simulink model "SF012A_HysCmp"  (R2013b)
settings: Solver=FixedStepDiscrete  StartTime=0.0  StopTime=1  FixedStep=.002  RelTol=1e-3
values from neighbouring files (symbols this model uses):
  ARCHGLBPRM_2MILLISEC_SEC_F32 = DataDict.Constant    [SF012A_HysCmp_DataDict.m]
  EPSILON_ULS_F32 = DataDict.Constant    [SF012A_HysCmp_DataDict.m]
  FLTINJ_HYSCMP_HYSCMPCMD = DataDict.Constant    [SF012A_HysCmp_DataDict.m]
  HysCmpAssiInpLim = DataDict.Calibration    [SF012A_HysCmp_DataDict.m]
  HysCmpOutpLim = DataDict.Calibration    [SF012A_HysCmp_DataDict.m]
  HysCmpRevGain = DataDict.Calibration    [SF012A_HysCmp_DataDict.m]
  HysCmpRiseX = DataDict.Calibration    [SF012A_HysCmp_DataDict.m]
  HysCmpRiseY = DataDict.Calibration    [SF012A_HysCmp_DataDict.m]
  HYSRISEYLIM_ULS_F32 = DataDict.Constant    [SF012A_HysCmp_DataDict.m]
  HYSSATNLOWLIM_HWNWTMTR_F32 = DataDict.Constant    [SF012A_HysCmp_DataDict.m]
  SysGlbPrmSysTqRat = DataDict.ImprtdCal    [SF012A_HysCmp_DataDict.m]
libraries: FixdToFloat x18, FloatToFixd x14, LnrIntrpn x12, NxtrAbslt x10, NxtrLim x8, Fil x6, NxtrSign x5, simulink x2, NxtrMath x1, BilnrIntrpnMplX x1, NxtrMax x1
(part 2 of 3)

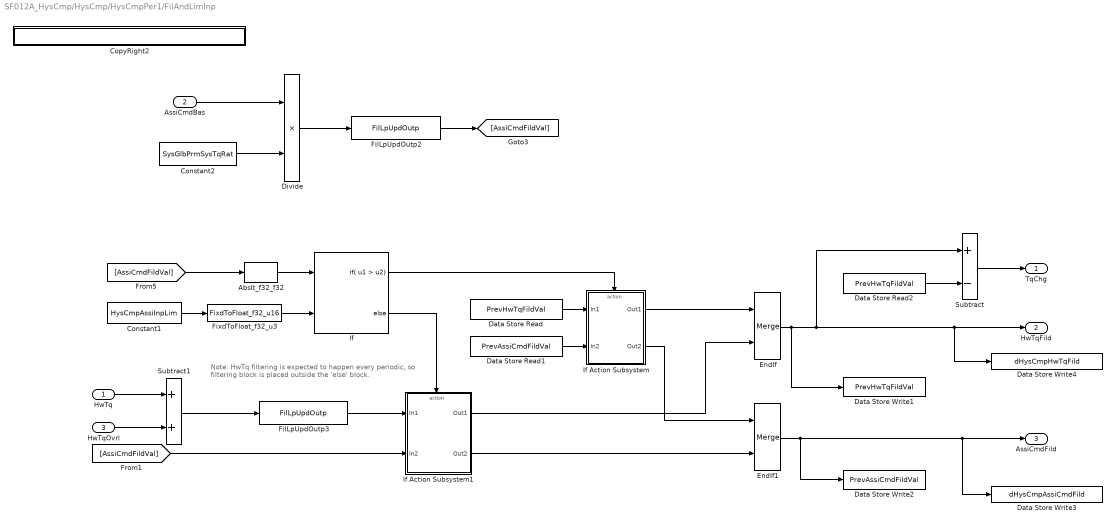
== system SF012A_HysCmp/HysCmp/HysCmpPer1/FilAndLimInp ==
  note: Note:
      | HwTq filtering is expected to happen every periodic, so filtering
      | block is placed outside the 'else' block.
  HwTq : Inport  RequirementInfo={'linktype_rmi_doors' '0000a52c (/E-STEER Core/SubSystem Specifications/Application Functions/SF012A Hysteresis Compensation)' '#SF012A_408' 'true' 'REQ:SF012A_408' '' } %GIDa_8595c692_04d6_4913_9dc2_51364eba2881
  AssiCmdBas : Inport  RequirementInfo={'linktype_rmi_doors' '0000a52c (/E-STEER Core/SubSystem Specifications/Application Functions/SF012A Hysteresis Compensation)' '#SF012A_409' 'true' 'REQ:SF012A_409' '' } %GIDa_dca39ed8_e3d9_4378_8b85_450d17c9d08c  Port=2
  HwTqOvrl : Inport  RequirementInfo={} %GIDa_e368a188_fa71_4a0d_b951_66914a67cd9f  Port=3
  Abslt_f32_f32 : NxtrAbslt/Abslt_f32_f32  RequirementInfo={'linktype_rmi_doors' '0000a52c (/E-STEER Core/SubSystem Specifications/Application Functions/SF012A Hysteresis Compensation)' '#SF012A_410' 'true' 'REQ:SF012A_410' '' ; 'linktype_rmi_doors' '0000a52c (/E-STEER Core/SubSystem Specifications/Application Functions/SF012A Hysteresis Compensation)' '#SF012A_411' 'true' 'REQ:SF012A_411' '' } %GIDa_f8d261e3_e868_420c_87ac_b2819908a7a3  SFunctionSpec=single y1 = Abslt_f32_f32(single u1)
      settings: AttributesFormatString=%<Name>
  Constant1 : Constant  RequirementInfo={'linktype_rmi_doors' '0000a52c (/E-STEER Core/SubSystem Specifications/Application Functions/SF012A Hysteresis Compensation)' '#SF012A_410' 'true' 'REQ:SF012A_410' '' ; 'linktype_rmi_doors' '0000a52c (/E-STEER Core/SubSystem Specifications/Application Functions/SF012A Hysteresis Compensation)' '#SF012A_411' 'true' 'REQ:SF012A_411' '' } %GIDa_864c3e61_20aa_4f8a_9abb_0e2225d86ec0  Value=HysCmpAssiInpLim
  Constant2 : Constant  RequirementInfo={'linktype_rmi_doors' '0000a52c (/E-STEER Core/SubSystem Specifications/Application Functions/SF012A Hysteresis Compensation)' '#SF012A_409' 'true' 'REQ:SF012A_409' '' } %GIDa_3b931750_8551_4b2a_8e8e_b917627f5aac  Value=SysGlbPrmSysTqRat
  CopyRight2 : Subsystem  Description=|  mask(Copyright Information){none=on}
      | Copyright info block.                                               
      |                                                                     
      | Place copyright information at the top of every subsystem in design.
      mask prompts: none "No parameters"
      mask help: Place copyright information at the top of every subsystem in design.
      mask Display:
      | NxtrConf = 'Nexteer Confidential';
      | 
      | sys = bdroot; %handle for the current model ("system")
      | first = get_param(sys,'Created');
      | if(isempty(first))
      |     first = datestr(now,'yyyy');
      | else
      |     first = first(end-3:end);  %year is last four digits
      | end
      | 
      | last = get_param(sys,'LastModifiedDate');
      | if isempty(last)
      |     last = datestr(now,'yyyy');
      | else
      |     last = last(end-3:end);
      | end
      | 
      | if strcmp(first,last)
      |     fprintf('%s -- Copyright %s Nexteer',NxtrConf,first)
      | else
      |     fprintf('%s -- %s%s- %s Nexteer',NxtrConf,char(169),first,last)
      | end
  Data Store Read : DataStoreRead  RequirementInfo={'linktype_rmi_doors' '0000a52c (/E-STEER Core/SubSystem Specifications/Application Functions/SF012A Hysteresis Compensation)' '#SF012A_410' 'true' 'REQ:SF012A_410' '' } %GIDa_fe2f0fc3_60a7_4f80_bf23_10f877f94ddf  DataStoreName=PrevHwTqFildVal
  Data Store Read1 : DataStoreRead  RequirementInfo={'linktype_rmi_doors' '0000a52c (/E-STEER Core/SubSystem Specifications/Application Functions/SF012A Hysteresis Compensation)' '#SF012A_411' 'true' 'REQ:SF012A_411' '' } %GIDa_d130b6b3_c629_46d9_812d_bdd319c1e1bb  DataStoreName=PrevAssiCmdFildVal
  Data Store Read2 : DataStoreRead  RequirementInfo={'linktype_rmi_doors' '0000a52c (/E-STEER Core/SubSystem Specifications/Application Functions/SF012A Hysteresis Compensation)' '#SF012A_413' 'true' 'REQ:SF012A_413' '' } %GIDa_ca0acc02_7cf7_474f_861e_05fd56275eb3  DataStoreName=PrevHwTqFildVal
  Data Store Write1 : DataStoreWrite  DataStoreName=PrevHwTqFildVal
  Data Store Write2 : DataStoreWrite  DataStoreName=PrevAssiCmdFildVal
  Data Store Write3 : DataStoreWrite  DataStoreName=dHysCmpAssiCmdFild
  Data Store Write4 : DataStoreWrite  DataStoreName=dHysCmpHwTqFild
  Divide : Product  RequirementInfo={'linktype_rmi_doors' '0000a52c (/E-STEER Core/SubSystem Specifications/Application Functions/SF012A Hysteresis Compensation)' '#SF012A_409' 'true' 'REQ:SF012A_409' '' } %GIDa_4801ace0_9cdb_47f1_b5c0_5f2abda0d87a
  EndIf : Merge
  EndIf1 : Merge
  FilLpUpdOutp2 : Fil/FilLpUpdOutp  RequirementInfo={'linktype_rmi_doors' '0000a52c (/E-STEER Core/SubSystem Specifications/Application Functions/SF012A Hysteresis Compensation)' '#SF012A_409' 'true' 'REQ:SF012A_409' '' } %GIDa_589584c9_b911_4f77_a83a_2b25e7b503c4  StVar=AssiCmdLpFil
      settings: AttributesFormatString=StVar: %<StVar>
  FilLpUpdOutp3 : Fil/FilLpUpdOutp  RequirementInfo={'linktype_rmi_doors' '0000a52c (/E-STEER Core/SubSystem Specifications/Application Functions/SF012A Hysteresis Compensation)' '#SF012A_408' 'true' 'REQ:SF012A_408' '' } %GIDa_7f89ab7f_0bec_4a90_b51d_fb631fff0f06  StVar=HwTqLpFil
      settings: AttributesFormatString=StVar: %<StVar>
  FixdToFloat_f32_u3 : FixdToFloat/FixdToFloat_f32_u16  RequirementInfo={'linktype_rmi_doors' '0000a52c (/E-STEER Core/SubSystem Specifications/Application Functions/SF012A Hysteresis Compensation)' '#SF012A_410' 'true' 'REQ:SF012A_410' '' ; 'linktype_rmi_doors' '0000a52c (/E-STEER Core/SubSystem Specifications/Application Functions/SF012A Hysteresis Compensation)' '#SF012A_411' 'true' 'REQ:SF012A_411' '' } %GIDa_0e35fb1f_9c33_4ae5_a8f9_936027a1a1ab  Param1=7
  If : If  RequirementInfo={'linktype_rmi_doors' '0000a52c (/E-STEER Core/SubSystem Specifications/Application Functions/SF012A Hysteresis Compensation)' '#SF012A_410' 'true' 'REQ:SF012A_410' '' ; 'linktype_rmi_doors' '0000a52c (/E-STEER Core/SubSystem Specifications/Application Functions/SF012A Hysteresis Compensation)' '#SF012A_411' 'true' 'REQ:SF012A_411' '' } %GIDa_f379a8d8_76cb_4a5a_bbf2_71e4ff64e958  NumInputs=2  IfExpression=u1 > u2
  If Action Subsystem : Subsystem  RequirementInfo={'linktype_rmi_doors' '0000a52c (/E-STEER Core/SubSystem Specifications/Application Functions/SF012A Hysteresis Compensation)' '#SF012A_410' 'true' 'REQ:SF012A_410' '' ; 'linktype_rmi_doors' '0000a52c (/E-STEER Core/SubSystem Specifications/Application Functions/SF012A Hysteresis Compensation)' '#SF012A_411' 'true' 'REQ:SF012A_411' '' } %GIDa_863f11eb_bed9_4787_8d86_71a303a919a1  TreatAsAtomicUnit=on
  If Action Subsystem1 : Subsystem  TreatAsAtomicUnit=on
  Subtract : Sum  RequirementInfo={'linktype_rmi_doors' '0000a52c (/E-STEER Core/SubSystem Specifications/Application Functions/SF012A Hysteresis Compensation)' '#SF012A_413' 'true' 'REQ:SF012A_413' '' } %GIDa_cc1a94d2_680b_41ba_bf31_9725f502d028  Inputs=+-  RndMeth=Zero
  Subtract1 : Sum  RequirementInfo="{'linktype_rmi_doors' '0000a52c (/E-STEER Core/SubSystem Specifications/Application Functions/SF012A Hysteresis Compensation)' '#SF012A_413' 'true' 'REQ:SF012A_413' '' ; 'linktype_rmi_doors' '0000a52c (/E-STEER Core/SubSystem Specifications/Application Functions/SF012A Hysteresis Compensation)' '#SF012A_408' 'true' 'REQ:  SF012A_408' '' } %GIDa_c73f89c5_e69d_4c2f_8313_728af91665f8"  RndMeth=Zero
  TqChg : Outport  RequirementInfo={'linktype_rmi_doors' '0000a52c (/E-STEER Core/SubSystem Specifications/Application Functions/SF012A Hysteresis Compensation)' '#SF012A_412' 'true' 'REQ:SF012A_412' '' } %GIDa_bba798dc_3c8f_457b_9533_3f83bd880396
  HwTqFild : Outport  Port=2
  AssiCmdFild : Outport  Port=3
  wires:
  FilLpUpdOutp2/1 -> [AssiCmdFildVal]
  Divide/1 -> FilLpUpdOutp2/1
  AssiCmdBas/1 -> Divide/1
  Constant2/1 -> Divide/2
  [AssiCmdFildVal] -> Abslt_f32_f32/1
  Abslt_f32_f32/1 -> If/1
  Constant1/1 -> FixdToFloat_f32_u3/1
  If/1 -> If Action Subsystem/Action
  If/2 -> If Action Subsystem1/Action
  [AssiCmdFildVal] -> If Action Subsystem1/2(In2)
  FilLpUpdOutp3/1 -> If Action Subsystem1/1(In1)
  If Action Subsystem1/1(Out1) -> EndIf/2
  If Action Subsystem/1(Out1) -> EndIf/1
  Data Store Read/1 -> If Action Subsystem/1(In1)
  Data Store Read1/1 -> If Action Subsystem/2(In2)
  If Action Subsystem/2(Out2) -> EndIf1/1
  If Action Subsystem1/2(Out2) -> EndIf1/2
  Subtract/1 -> TqChg/1
  EndIf/1 -> Data Store Write1/1, Data Store Write4/1, HwTqFild/1, Subtract/1
  Data Store Read2/1 -> Subtract/2
  EndIf1/1 -> Data Store Write3/1, AssiCmdFild/1, Data Store Write2/1
  FixdToFloat_f32_u3/1 -> If/2
  Subtract1/1 -> FilLpUpdOutp3/1
  HwTq/1 -> Subtract1/1
  HwTqOvrl/1 -> Subtract1/2

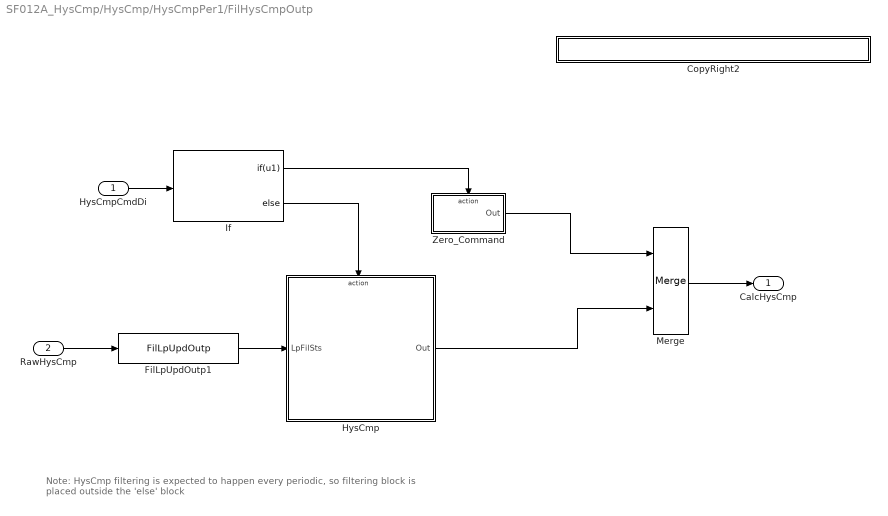
== system SF012A_HysCmp/HysCmp/HysCmpPer1/FilHysCmpOutp ==
  note: Note:
      | HysCmp filtering is expected to happen every periodic, so filtering block is placed
      | outside the 'else' block
  HysCmpCmdDi : Inport  RequirementInfo={'linktype_rmi_doors' '0000a52c (/E-STEER Core/SubSystem Specifications/Application Functions/SF012A Hysteresis Compensation)' '#SF012A_459' 'true' 'REQ:SF012A_459' '' } %GIDa_23db5d3c_8a57_4504_bba3_7c9578b077b2
  RawHysCmp : Inport  RequirementInfo={'linktype_rmi_doors' '0000a52c (/E-STEER Core/SubSystem Specifications/Application Functions/SF012A Hysteresis Compensation)' '#SF012A_457' 'true' 'REQ:SF012A_457' '' } %GIDa_195e1d1d_69bd_4591_afc7_b0c2a9192583  Port=2
  CopyRight2 : Subsystem  Description=|  mask(Copyright Information){none=on}
      | Copyright info block.                                               
      |                                                                     
      | Place copyright information at the top of every subsystem in design.
      mask prompts: none "No parameters"
      mask help: Place copyright information at the top of every subsystem in design.
      mask Display:
      | NxtrConf = 'Nexteer Confidential';
      | 
      | sys = bdroot; %handle for the current model ("system")
      | first = get_param(sys,'Created');
      | if(isempty(first))
      |     first = datestr(now,'yyyy');
      | else
      |     first = first(end-3:end);  %year is last four digits
      | end
      | 
      | last = get_param(sys,'LastModifiedDate');
      | if isempty(last)
      |     last = datestr(now,'yyyy');
      | else
      |     last = last(end-3:end);
      | end
      | 
      | if strcmp(first,last)
      |     fprintf('%s -- Copyright %s Nexteer',NxtrConf,first)
      | else
      |     fprintf('%s -- %s%s- %s Nexteer',NxtrConf,char(169),first,last)
      | end
  FilLpUpdOutp1 : Fil/FilLpUpdOutp  RequirementInfo={'linktype_rmi_doors' '0000a52c (/E-STEER Core/SubSystem Specifications/Application Functions/SF012A Hysteresis Compensation)' '#SF012A_457' 'true' 'REQ:SF012A_457' '' } %GIDa_9e2ef691_d79e_479f_a90d_387920e70bae  StVar=FinalOutpLpFil
      settings: AttributesFormatString=StVar: %<StVar>
  HysCmp : Subsystem  RequirementInfo={} %GIDa_95224ba3_d373_47aa_9e2d_c8f1beaf79f1  TreatAsAtomicUnit=on
  If : If  RequirementInfo={'linktype_rmi_doors' '0000a52c (/E-STEER Core/SubSystem Specifications/Application Functions/SF012A Hysteresis Compensation)' '#SF012A_459' 'true' 'REQ:SF012A_459' '' } %GIDa_94a310f4_6e32_4cd6_8e0d_2a7931f46409  IfExpression=u1
  Merge : Merge
  Zero_Command : Subsystem  RequirementInfo={'linktype_rmi_doors' '0000a52c (/E-STEER Core/SubSystem Specifications/Application Functions/SF012A Hysteresis Compensation)' '#SF012A_459' 'true' 'REQ:SF012A_459' '' } %GIDa_7dfea39b_76f9_4579_a42d_48172b08e8b5  TreatAsAtomicUnit=on
  CalcHysCmp : Outport
  wires:
  HysCmp/1(Out) -> Merge/2
  If/1 -> Zero_Command/Action
  If/2 -> HysCmp/Action
  HysCmpCmdDi/1 -> If/1
  Zero_Command/1(Out) -> Merge/1
  Merge/1 -> CalcHysCmp/1
  RawHysCmp/1 -> FilLpUpdOutp1/1
  FilLpUpdOutp1/1 -> HysCmp/1(LpFilSts)

== system SF012A_HysCmp/HysCmp/HysCmpPer1/FltInj - Sim ==
  note: Inport #2 must be Constant
  note: EA4.x Fault Injection
  note: This block requires no modification by FDD author.
      |
      | This block does not actually simulate any fault injection.  It is simply a pass-thru.
      |
      | The port (#2) simply terminates its signal, but we are trying to force the FDD author
      | to properly use the Constant in FDD model.
  HysCmp : Inport
  FltInjCon : Inport  Port=2
  CopyRight2 : Subsystem  Description=|  mask(Copyright Information){none=on}
      | Copyright info block.                                               
      |                                                                     
      | Place copyright information at the top of every subsystem in design.
      mask prompts: none "No parameters"
      mask help: Place copyright information at the top of every subsystem in design.
      mask Display:
      | NxtrConf = 'Nexteer Confidential';
      | 
      | sys = bdroot; %handle for the current model ("system")
      | first = get_param(sys,'Created');
      | if(isempty(first))
      |     first = datestr(now,'yyyy');
      | else
      |     first = first(end-3:end);  %year is last four digits
      | end
      | 
      | last = get_param(sys,'LastModifiedDate');
      | if isempty(last)
      |     last = datestr(now,'yyyy');
      | else
      |     last = last(end-3:end);
      | end
      | 
      | if strcmp(first,last)
      |     fprintf('%s -- Copyright %s Nexteer',NxtrConf,first)
      | else
      |     fprintf('%s -- %s%s- %s Nexteer',NxtrConf,char(169),first,last)
      | end
  Terminator : Terminator
  Outp : Outport
  wires:
  FltInjCon/1 -> Terminator/1
  HysCmp/1 -> Outp/1

== system SF012A_HysCmp/HysCmp/HysCmpPer1/CalcAvlCmp/CopyRight2 ==

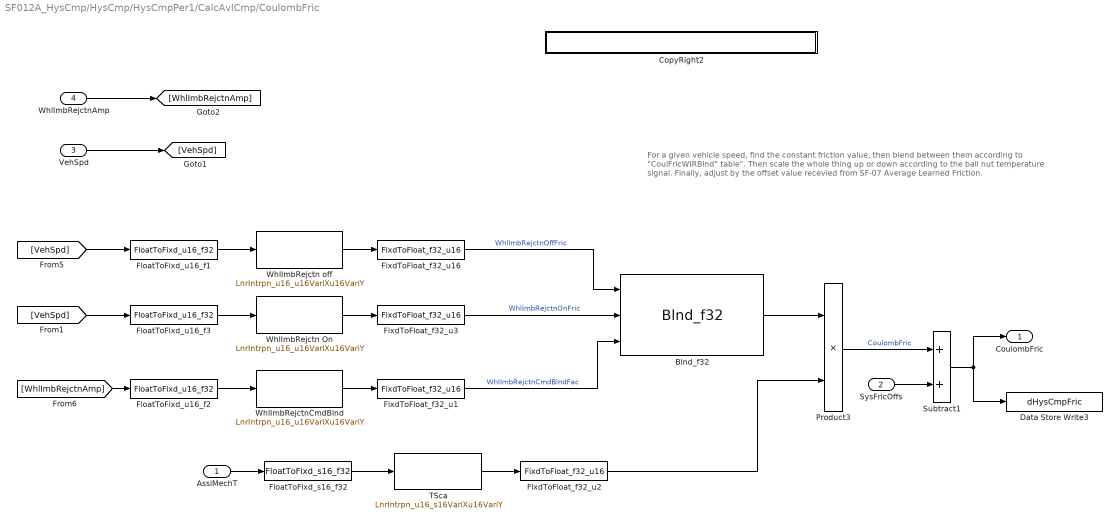
== system SF012A_HysCmp/HysCmp/HysCmpPer1/CalcAvlCmp/CoulombFric ==
  note: For a given vehicle speed, find the constant friction value, then blend between them
      | according to "CoulFricWIRBlnd" table".
      |
      | Then scale the whole thing up or down according to the ball nut temperature signal.
      |
      | Finally, adjust by the offset value recevied from SF-07 Average Learned Friction.
  AssiMechT : Inport  RequirementInfo={'linktype_rmi_doors' '0000a52c (/E-STEER Core/SubSystem Specifications/Application Functions/SF012A Hysteresis Compensation)' '#SF012A_449' 'true' 'REQ:SF012A_449' '' } %GIDa_99e06030_f9cc_4e47_87aa_b53708a11645
  SysFricOffs : Inport  RequirementInfo={'linktype_rmi_doors' '0000a52c (/E-STEER Core/SubSystem Specifications/Application Functions/SF012A Hysteresis Compensation)' '#SF012A_450' 'true' 'REQ:SF012A_450' '' } %GIDa_ac543b49_7806_48b8_bba0_d91827b9781a  Port=2
  VehSpd : Inport  Port=3
  WhlImbRejctnAmp : Inport  Port=4
  Blnd_f32 : NxtrMath/Blnd_f32  RequirementInfo={'linktype_rmi_doors' '0000a52c (/E-STEER Core/SubSystem Specifications/Application Functions/SF012A Hysteresis Compensation)' '#SF012A_448' 'true' 'REQ:SF012A_448' '' } %GIDa_bbdb4f9c_3bc2_498f_af71_2f49518b1990  SFunctionSpec=single y1 = Blnd_f32(single u1, single u2, single u3)  Parameter3=on
      settings: AttributesFormatString=%<Name>
  CopyRight2 : Subsystem  Description=|  mask(Copyright Information){none=on}
      | Copyright info block.                                               
      |                                                                     
      | Place copyright information at the top of every subsystem in design.
      mask prompts: none "No parameters"
      mask help: Place copyright information at the top of every subsystem in design.
      mask Display:
      | NxtrConf = 'Nexteer Confidential';
      | 
      | sys = bdroot; %handle for the current model ("system")
      | first = get_param(sys,'Created');
      | if(isempty(first))
      |     first = datestr(now,'yyyy');
      | else
      |     first = first(end-3:end);  %year is last four digits
      | end
      | 
      | last = get_param(sys,'LastModifiedDate');
      | if isempty(last)
      |     last = datestr(now,'yyyy');
      | else
      |     last = last(end-3:end);
      | end
      | 
      | if strcmp(first,last)
      |     fprintf('%s -- Copyright %s Nexteer',NxtrConf,first)
      | else
      |     fprintf('%s -- %s%s- %s Nexteer',NxtrConf,char(169),first,last)
      | end
  Data Store Write3 : DataStoreWrite  RequirementInfo={'linktype_rmi_doors' '0000a52c (/E-STEER Core/SubSystem Specifications/Application Functions/SF012A Hysteresis Compensation)' '#SF012A_450' 'true' 'REQ:SF012A_450' '' } %GIDa_6d45951a_d82c_43e3_9e30_495c6992e5fa  DataStoreName=dHysCmpFric
  FixdToFloat_f32_u1 : FixdToFloat/FixdToFloat_f32_u16  RequirementInfo={'linktype_rmi_doors' '0000a52c (/E-STEER Core/SubSystem Specifications/Application Functions/SF012A Hysteresis Compensation)' '#SF012A_447' 'true' 'REQ:SF012A_447' '' } %GIDa_6923d4d2_9d71_4e52_940a_040d870df5d3  Param1=14
  FixdToFloat_f32_u16 : FixdToFloat/FixdToFloat_f32_u16  RequirementInfo={'linktype_rmi_doors' '0000a52c (/E-STEER Core/SubSystem Specifications/Application Functions/SF012A Hysteresis Compensation)' '#SF012A_445' 'true' 'REQ:SF012A_445' '' } %GIDa_30d19d68_5b37_4b98_9d06_6ac023f5c633  Param1=7
  FixdToFloat_f32_u2 : FixdToFloat/FixdToFloat_f32_u16  RequirementInfo={'linktype_rmi_doors' '0000a52c (/E-STEER Core/SubSystem Specifications/Application Functions/SF012A Hysteresis Compensation)' '#SF012A_449' 'true' 'REQ:SF012A_449' '' } %GIDa_e9926a9e_58d8_4e0f_b85f_c8f228f08a51  Param1=7
  FixdToFloat_f32_u3 : FixdToFloat/FixdToFloat_f32_u16  RequirementInfo={'linktype_rmi_doors' '0000a52c (/E-STEER Core/SubSystem Specifications/Application Functions/SF012A Hysteresis Compensation)' '#SF012A_446' 'true' 'REQ:SF012A_446' '' } %GIDa_029b97c1_98e5_43d6_8bb2_f228e7ba74a0  Param1=7
  FloatToFixd_s16_f32 : FloatToFixd/FloatToFixd_s16_f32  RequirementInfo={'linktype_rmi_doors' '0000a52c (/E-STEER Core/SubSystem Specifications/Application Functions/SF012A Hysteresis Compensation)' '#SF012A_449' 'true' 'REQ:SF012A_449' '' } %GIDa_ed7de31a_137c_4cee_b956_f1a1d053aab7  Param1=1
  FloatToFixd_u16_f1 : FloatToFixd/FloatToFixd_u16_f32  RequirementInfo={'linktype_rmi_doors' '0000a52c (/E-STEER Core/SubSystem Specifications/Application Functions/SF012A Hysteresis Compensation)' '#SF012A_445' 'true' 'REQ:SF012A_445' '' } %GIDa_d5c90da9_066a_4c50_b363_eaa13c485fc7  Param1=7
  FloatToFixd_u16_f2 : FloatToFixd/FloatToFixd_u16_f32  RequirementInfo={'linktype_rmi_doors' '0000a52c (/E-STEER Core/SubSystem Specifications/Application Functions/SF012A Hysteresis Compensation)' '#SF012A_447' 'true' 'REQ:SF012A_447' '' } %GIDa_1211a0db_eafe_40ef_b441_39a05294fb9a  Param1=8
  FloatToFixd_u16_f3 : FloatToFixd/FloatToFixd_u16_f32  RequirementInfo={'linktype_rmi_doors' '0000a52c (/E-STEER Core/SubSystem Specifications/Application Functions/SF012A Hysteresis Compensation)' '#SF012A_446' 'true' 'REQ:SF012A_446' '' } %GIDa_1e28c5e9_2e43_4a13_a086_2e913b05aeaf  Param1=7
  Product3 : Product  RequirementInfo={'linktype_rmi_doors' '0000a52c (/E-STEER Core/SubSystem Specifications/Application Functions/SF012A Hysteresis Compensation)' '#SF012A_449' 'true' 'REQ:SF012A_449' '' } %GIDa_88ab9335_d857_42a9_939b_fda1c9a4430d  RndMeth=Zero
  Subtract1 : Sum  RequirementInfo={'linktype_rmi_doors' '0000a52c (/E-STEER Core/SubSystem Specifications/Application Functions/SF012A Hysteresis Compensation)' '#SF012A_450' 'true' 'REQ:SF012A_450' '' } %GIDa_00ed35e3_2a2d_45e4_ac36_bcf0983ee021
  TSca : LnrIntrpn/LnrIntrpn_u16_s16VariXu16VariY  RequirementInfo={'linktype_rmi_doors' '0000a52c (/E-STEER Core/SubSystem Specifications/Application Functions/SF012A Hysteresis Compensation)' '#SF012A_449' 'true' 'REQ:SF012A_449' '' } %GIDa_1507d625_50ab_420f_903c_b0ff65633902  XTbl=HysCmpFricTScaX  YTbl=HysCmpFricTScaY
      settings: AttributesFormatString=Lnr ( s16VariX , u16VariY )
  WhlImbRejctn On : LnrIntrpn/LnrIntrpn_u16_u16VariXu16VariY  RequirementInfo={'linktype_rmi_doors' '0000a52c (/E-STEER Core/SubSystem Specifications/Application Functions/SF012A Hysteresis Compensation)' '#SF012A_446' 'true' 'REQ:SF012A_446' '' } %GIDa_3da3a5f4_48bb_4b0e_875e_441bf1ad5aca  XTbl=SysGlbPrmVehSpdBilnrSeln  YTbl=HysCmpFricWhlImbRejctnOnY
      settings: AttributesFormatString=Lnr ( u16VariX , u16VariY )
  WhlImbRejctn off : LnrIntrpn/LnrIntrpn_u16_u16VariXu16VariY  RequirementInfo={'linktype_rmi_doors' '0000a52c (/E-STEER Core/SubSystem Specifications/Application Functions/SF012A Hysteresis Compensation)' '#SF012A_445' 'true' 'REQ:SF012A_445' '' } %GIDa_4a3d582a_5707_4fce_81eb_d8533e9ef487  XTbl=SysGlbPrmVehSpdBilnrSeln  YTbl=HysCmpFricWhlImbRejctnOffY
      settings: AttributesFormatString=Lnr ( u16VariX , u16VariY )
  WhlImbRejctnCmdBlnd : LnrIntrpn/LnrIntrpn_u16_u16VariXu16VariY  RequirementInfo={'linktype_rmi_doors' '0000a52c (/E-STEER Core/SubSystem Specifications/Application Functions/SF012A Hysteresis Compensation)' '#SF012A_447' 'true' 'REQ:SF012A_447' '' } %GIDa_665c52af_bd47_42fe_9c42_9c84618a0bfd  XTbl=HysCmpFricWhlImbRejctnBlndX  YTbl=HysCmpFricWhlImbRejctnBlndY
      settings: AttributesFormatString=Lnr ( u16VariX , u16VariY )
  CoulombFric : Outport  RequirementInfo={'linktype_rmi_doors' '0000a52c (/E-STEER Core/SubSystem Specifications/Application Functions/SF012A Hysteresis Compensation)' '#SF012A_450' 'true' 'REQ:SF012A_450' '' } %GIDa_05ee5a21_5232_467a_82a3_6197e6a6ac48
  wires:
  AssiMechT/1 -> FloatToFixd_s16_f32/1
  SysFricOffs/1 -> Subtract1/2
  VehSpd/1 -> [VehSpd]
  WhlImbRejctnAmp/1 -> [WhlImbRejctnAmp]
  FloatToFixd_s16_f32/1 -> TSca/1
  TSca/1 -> FixdToFloat_f32_u2/1
  FixdToFloat_f32_u2/1 -> Product3/2
  Product3/1 -> Subtract1/1  "CoulombFric"
  Subtract1/1 -> Data Store Write3/1, CoulombFric/1
  [VehSpd] -> FloatToFixd_u16_f1/1
  FloatToFixd_u16_f1/1 -> WhlImbRejctn off/1
  WhlImbRejctnCmdBlnd/1 -> FixdToFloat_f32_u1/1
  [WhlImbRejctnAmp] -> FloatToFixd_u16_f2/1
  FixdToFloat_f32_u16/1 -> Blnd_f32/1  "WhlImbRejctnOffFric"
  FloatToFixd_u16_f2/1 -> WhlImbRejctnCmdBlnd/1
  FixdToFloat_f32_u1/1 -> Blnd_f32/3  "WhlImbRejctnCmdBlndFac"
  [VehSpd] -> FloatToFixd_u16_f3/1
  FloatToFixd_u16_f3/1 -> WhlImbRejctn On/1
  FixdToFloat_f32_u3/1 -> Blnd_f32/2  "WhlImbRejctnOnFric"
  WhlImbRejctn On/1 -> FixdToFloat_f32_u3/1
  WhlImbRejctn off/1 -> FixdToFloat_f32_u16/1
  Blnd_f32/1 -> Product3/1

== system SF012A_HysCmp/HysCmp/HysCmpPer1/CalcRiseFac/CopyRight2 ==

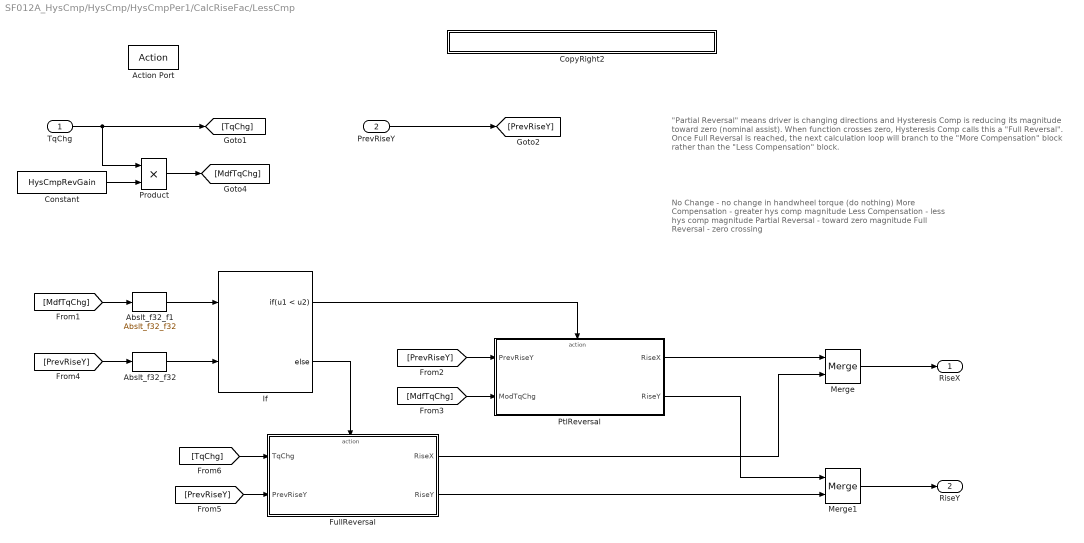
== system SF012A_HysCmp/HysCmp/HysCmpPer1/CalcRiseFac/LessCmp ==
  note: No Change                    - no change in handwheel torque (do nothing)
      |
      | More Compensation     - greater hys comp magnitude
      |
      | Less Compensation     - less hys comp magnitude
      |        Partial Reversal          - toward zero magnitude
      |        Full Reversal               - zero crossing
  note: "Partial Reversal" means driver is changing directions and Hysteresis Comp is reducing its magnitude toward
      | zero (nominal assist).  When function crosses zero, Hysteresis Comp calls this a "Full Reversal".  Once
      | Full Reversal is reached, the next calculation loop will branch to the "More Compensation" block rather
      | than the "Less Compensation" block.
  TqChg : Inport  RequirementInfo={'linktype_rmi_doors' '0000a52c (/E-STEER Core/SubSystem Specifications/Application Functions/SF012A Hysteresis Compensation)' '#SF012A_427' 'true' 'REQ:SF012A_427' '' } %GIDa_99dd5ad1_f987_430b_9292_ba160c7a64e2
  PrevRiseY : Inport  Port=2
  Action Port : ActionPort  ActionType=else
  Abslt_f32_f1 : NxtrAbslt/Abslt_f32_f32  RequirementInfo={'linktype_rmi_doors' '0000a52c (/E-STEER Core/SubSystem Specifications/Application Functions/SF012A Hysteresis Compensation)' '#SF012A_430' 'true' 'REQ:SF012A_430' '' ; 'linktype_rmi_doors' '0000a52c (/E-STEER Core/SubSystem Specifications/Application Functions/SF012A Hysteresis Compensation)' '#SF012A_434' 'true' 'REQ:SF012A_434' '' } %GIDa_cb35d4e0_44c4_4ae0_8e61_ff94531bb974  SFunctionSpec=single y1 = Abslt_f32_f32(single u1)
      settings: AttributesFormatString=%<Name>
  Abslt_f32_f32 : NxtrAbslt/Abslt_f32_f32  RequirementInfo={'linktype_rmi_doors' '0000a52c (/E-STEER Core/SubSystem Specifications/Application Functions/SF012A Hysteresis Compensation)' '#SF012A_430' 'true' 'REQ:SF012A_430' '' ; 'linktype_rmi_doors' '0000a52c (/E-STEER Core/SubSystem Specifications/Application Functions/SF012A Hysteresis Compensation)' '#SF012A_434' 'true' 'REQ:SF012A_434' '' } %GIDa_784ab8b6_4235_4986_832e_173db3fc1314  SFunctionSpec=single y1 = Abslt_f32_f32(single u1)
      settings: AttributesFormatString=%<Name>
  Constant : Constant  RequirementInfo={'linktype_rmi_doors' '0000a52c (/E-STEER Core/SubSystem Specifications/Application Functions/SF012A Hysteresis Compensation)' '#SF012A_427' 'true' 'REQ:SF012A_427' '' } %GIDa_15f6df37_2f5f_4b2b_9a59_ced4ab5b144b  Value=HysCmpRevGain
  CopyRight2 : Subsystem  Description=|  mask(Copyright Information){none=on}
      | Copyright info block.                                               
      |                                                                     
      | Place copyright information at the top of every subsystem in design.
      mask prompts: none "No parameters"
      mask help: Place copyright information at the top of every subsystem in design.
      mask Display:
      | NxtrConf = 'Nexteer Confidential';
      | 
      | sys = bdroot; %handle for the current model ("system")
      | first = get_param(sys,'Created');
      | if(isempty(first))
      |     first = datestr(now,'yyyy');
      | else
      |     first = first(end-3:end);  %year is last four digits
      | end
      | 
      | last = get_param(sys,'LastModifiedDate');
      | if isempty(last)
      |     last = datestr(now,'yyyy');
      | else
      |     last = last(end-3:end);
      | end
      | 
      | if strcmp(first,last)
      |     fprintf('%s -- Copyright %s Nexteer',NxtrConf,first)
      | else
      |     fprintf('%s -- %s%s- %s Nexteer',NxtrConf,char(169),first,last)
      | end
  FullReversal : Subsystem  RequirementInfo={'linktype_rmi_doors' '0000a52c (/E-STEER Core/SubSystem Specifications/Application Functions/SF012A Hysteresis Compensation)' '#SF012A_433' 'true' 'REQ:SF012A_433' '' } %GIDa_ec6c7e68_d561_42f7_b642_302ca9573c52  TreatAsAtomicUnit=on
  If : If  RequirementInfo={'linktype_rmi_doors' '0000a52c (/E-STEER Core/SubSystem Specifications/Application Functions/SF012A Hysteresis Compensation)' '#SF012A_430' 'true' 'REQ:SF012A_430' '' ; 'linktype_rmi_doors' '0000a52c (/E-STEER Core/SubSystem Specifications/Application Functions/SF012A Hysteresis Compensation)' '#SF012A_434' 'true' 'REQ:SF012A_434' '' } %GIDa_cd0f389b_ef71_46b6_bbe9_7b7e3cd1952a  NumInputs=2  IfExpression=u1 < u2
  Merge : Merge
  Merge1 : Merge
  Product : Product  RequirementInfo={'linktype_rmi_doors' '0000a52c (/E-STEER Core/SubSystem Specifications/Application Functions/SF012A Hysteresis Compensation)' '#SF012A_427' 'true' 'REQ:SF012A_427' '' } %GIDa_7ff331fe_9280_41b2_bd53_ab63015d89f2  RndMeth=Zero
  PtlReversal : Subsystem  RequirementInfo={'linktype_rmi_doors' '0000a52c (/E-STEER Core/SubSystem Specifications/Application Functions/SF012A Hysteresis Compensation)' '#SF012A_429' 'true' 'REQ:SF012A_429' '' } %GIDa_b76a0e39_afe4_4599_8d0e_a01df819218b  TreatAsAtomicUnit=on
  RiseX : Outport
  RiseY : Outport  Port=2
  wires:
  TqChg/1 -> Product/1, [TqChg]
  PrevRiseY/1 -> [PrevRiseY]
  Product/1 -> [MdfTqChg]
  [PrevRiseY] -> Abslt_f32_f32/1
  Abslt_f32_f32/1 -> If/2
  [MdfTqChg] -> Abslt_f32_f1/1
  Abslt_f32_f1/1 -> If/1
  If/1 -> PtlReversal/Action
  If/2 -> FullReversal/Action
  [PrevRiseY] -> PtlReversal/1(PrevRiseY)
  [MdfTqChg] -> PtlReversal/2(ModTqChg)
  [PrevRiseY] -> FullReversal/2(PrevRiseY)
  [TqChg] -> FullReversal/1(TqChg)
  PtlReversal/1(RiseX) -> Merge/1
  PtlReversal/2(RiseY) -> Merge1/1
  Merge/1 -> RiseX/1
  Merge1/1 -> RiseY/1
  FullReversal/1(RiseX) -> Merge/2
  FullReversal/2(RiseY) -> Merge1/2
  Constant/1 -> Product/2

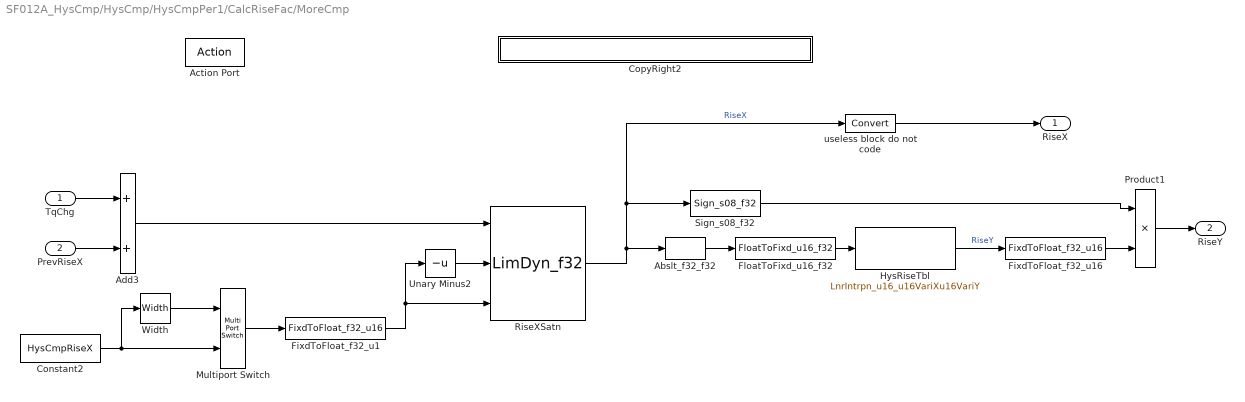
== system SF012A_HysCmp/HysCmp/HysCmpPer1/CalcRiseFac/MoreCmp ==
  TqChg : Inport  RequirementInfo={'linktype_rmi_doors' '0000a52c (/E-STEER Core/SubSystem Specifications/Application Functions/SF012A Hysteresis Compensation)' '#SF012A_423' 'true' 'REQ:SF012A_423' '' } %GIDa_dcd955d8_e60c_4b32_934a_4c581dd85aa1
  PrevRiseX : Inport  RequirementInfo={'linktype_rmi_doors' '0000a52c (/E-STEER Core/SubSystem Specifications/Application Functions/SF012A Hysteresis Compensation)' '#SF012A_423' 'true' 'REQ:SF012A_423' '' } %GIDa_087dae41_8153_4d25_bd8f_934a3a8ff619  Port=2
  Action Port : ActionPort  ActionType=elseif
  Abslt_f32_f32 : NxtrAbslt/Abslt_f32_f32  RequirementInfo={'linktype_rmi_doors' '0000a52c (/E-STEER Core/SubSystem Specifications/Application Functions/SF012A Hysteresis Compensation)' '#SF012A_425' 'true' 'REQ:SF012A_425' '' } %GIDa_32c7f8a9_d2f9_4a69_a73d_851dc6a3d9da  SFunctionSpec=single y1 = Abslt_f32_f32(single u1)
      settings: AttributesFormatString=%<Name>
  Add3 : Sum  RequirementInfo={'linktype_rmi_doors' '0000a52c (/E-STEER Core/SubSystem Specifications/Application Functions/SF012A Hysteresis Compensation)' '#SF012A_423' 'true' 'REQ:SF012A_423' '' } %GIDa_d9459225_db2d_4211_a8e1_86c473c2aa48  RndMeth=Zero
  Constant2 : Constant  RequirementInfo={'linktype_rmi_doors' '0000a52c (/E-STEER Core/SubSystem Specifications/Application Functions/SF012A Hysteresis Compensation)' '#SF012A_424' 'true' 'REQ:SF012A_424' '' } %GIDa_d2b201c3_0390_42ff_a153_be580eaf717d  Value=HysCmpRiseX
  CopyRight2 : Subsystem  Description=|  mask(Copyright Information){none=on}
      | Copyright info block.                                               
      |                                                                     
      | Place copyright information at the top of every subsystem in design.
      mask prompts: none "No parameters"
      mask help: Place copyright information at the top of every subsystem in design.
      mask Display:
      | NxtrConf = 'Nexteer Confidential';
      | 
      | sys = bdroot; %handle for the current model ("system")
      | first = get_param(sys,'Created');
      | if(isempty(first))
      |     first = datestr(now,'yyyy');
      | else
      |     first = first(end-3:end);  %year is last four digits
      | end
      | 
      | last = get_param(sys,'LastModifiedDate');
      | if isempty(last)
      |     last = datestr(now,'yyyy');
      | else
      |     last = last(end-3:end);
      | end
      | 
      | if strcmp(first,last)
      |     fprintf('%s -- Copyright %s Nexteer',NxtrConf,first)
      | else
      |     fprintf('%s -- %s%s- %s Nexteer',NxtrConf,char(169),first,last)
      | end
  FixdToFloat_f32_u1 : FixdToFloat/FixdToFloat_f32_u16  RequirementInfo={'linktype_rmi_doors' '0000a52c (/E-STEER Core/SubSystem Specifications/Application Functions/SF012A Hysteresis Compensation)' '#SF012A_424' 'true' 'REQ:SF012A_424' '' } %GIDa_ba8154cf_569f_4ec9_bec9_04076a244e06  Param1=14
  FixdToFloat_f32_u16 : FixdToFloat/FixdToFloat_f32_u16  RequirementInfo={'linktype_rmi_doors' '0000a52c (/E-STEER Core/SubSystem Specifications/Application Functions/SF012A Hysteresis Compensation)' '#SF012A_425' 'true' 'REQ:SF012A_425' '' } %GIDa_9bb57ca1_48e0_4f1a_9eca_c1d1a458fd1d  Param1=14
  FloatToFixd_u16_f32 : FloatToFixd/FloatToFixd_u16_f32  RequirementInfo={'linktype_rmi_doors' '0000a52c (/E-STEER Core/SubSystem Specifications/Application Functions/SF012A Hysteresis Compensation)' '#SF012A_425' 'true' 'REQ:SF012A_425' '' } %GIDa_f4755063_919f_46d9_8399_73ec98d9ae0d  Param1=14
  HysRiseTbl : LnrIntrpn/LnrIntrpn_u16_u16VariXu16VariY  RequirementInfo={'linktype_rmi_doors' '0000a52c (/E-STEER Core/SubSystem Specifications/Application Functions/SF012A Hysteresis Compensation)' '#SF012A_425' 'true' 'REQ:SF012A_425' '' } %GIDa_7e3a87f1_77a6_41da_8277_b0453ebcfa14  XTbl=HysCmpRiseX  YTbl=HysCmpRiseY
      settings: AttributesFormatString=Lnr ( u16VariX , u16VariY )
  Multiport Switch : MultiPortSwitch  RequirementInfo={'linktype_rmi_doors' '0000a52c (/E-STEER Core/SubSystem Specifications/Application Functions/SF012A Hysteresis Compensation)' '#SF012A_424' 'true' 'REQ:SF012A_424' '' } %GIDa_61a32efe_55fc_478c_b9d1_e4654c50a2e9  Inputs=1
  Product1 : Product  RequirementInfo={'linktype_rmi_doors' '0000a52c (/E-STEER Core/SubSystem Specifications/Application Functions/SF012A Hysteresis Compensation)' '#SF012A_425' 'true' 'REQ:SF012A_425' '' } %GIDa_784fab1f_e8ed_4e00_912d_e356e165dc4a  RndMeth=Zero
  RiseXSatn : NxtrLim/LimDyn_f32  RequirementInfo={'linktype_rmi_doors' '0000a52c (/E-STEER Core/SubSystem Specifications/Application Functions/SF012A Hysteresis Compensation)' '#SF012A_424' 'true' 'REQ:SF012A_424' '' } %GIDa_fc5089ee_ade2_4851_9608_4e2c221f2b41
  Sign_s08_f32 : NxtrSign/Sign_s08_f32  RequirementInfo={'linktype_rmi_doors' '0000a52c (/E-STEER Core/SubSystem Specifications/Application Functions/SF012A Hysteresis Compensation)' '#SF012A_425' 'true' 'REQ:SF012A_425' '' } %GIDa_75914151_b87b_403f_b5d7_9e430c415640  SFunctionSpec=int8 y1 = Sign_s08_f32(single u1)
  Unary Minus2 : UnaryMinus  RequirementInfo={'linktype_rmi_doors' '0000a52c (/E-STEER Core/SubSystem Specifications/Application Functions/SF012A Hysteresis Compensation)' '#SF012A_424' 'true' 'REQ:SF012A_424' '' } %GIDa_40aeac15_ec2a_4bb3_84ef_45980d7d55b1
  Width : Width  RequirementInfo={'linktype_rmi_doors' '0000a52c (/E-STEER Core/SubSystem Specifications/Application Functions/SF012A Hysteresis Compensation)' '#SF012A_424' 'true' 'REQ:SF012A_424' '' } %GIDa_dd860dde_6eef_4e41_9378_439bb9d42621  DataType=uint16
  useless block do not code : DataTypeConversion
  RiseX : Outport
  RiseY : Outport  Port=2
  wires:
  PrevRiseX/1 -> Add3/2
  TqChg/1 -> Add3/1
  Add3/1 -> RiseXSatn/1
  Constant2/1 -> Multiport Switch/2, Width/1
  Unary Minus2/1 -> RiseXSatn/2
  RiseXSatn/1 -> Sign_s08_f32/1, useless block do not code/1, Abslt_f32_f32/1  "RiseX"
  Sign_s08_f32/1 -> Product1/1
  Abslt_f32_f32/1 -> FloatToFixd_u16_f32/1
  HysRiseTbl/1 -> FixdToFloat_f32_u16/1  "RiseY"
  Product1/1 -> RiseY/1
  FloatToFixd_u16_f32/1 -> HysRiseTbl/1
  FixdToFloat_f32_u16/1 -> Product1/2
  Width/1 -> Multiport Switch/1
  Multiport Switch/1 -> FixdToFloat_f32_u1/1
  FixdToFloat_f32_u1/1 -> Unary Minus2/1, RiseXSatn/3
  useless block do not code/1 -> RiseX/1

== system SF012A_HysCmp/HysCmp/HysCmpPer1/CalcRiseFac/NoChg ==
  PrevRiseX : Inport
  PrevRiseY : Inport  Port=2
  Action Port : ActionPort  ActionType=then
  CopyRight2 : Subsystem  Description=|  mask(Copyright Information){none=on}
      | Copyright info block.                                               
      |                                                                     
      | Place copyright information at the top of every subsystem in design.
      mask prompts: none "No parameters"
      mask help: Place copyright information at the top of every subsystem in design.
      mask Display:
      | NxtrConf = 'Nexteer Confidential';
      | 
      | sys = bdroot; %handle for the current model ("system")
      | first = get_param(sys,'Created');
      | if(isempty(first))
      |     first = datestr(now,'yyyy');
      | else
      |     first = first(end-3:end);  %year is last four digits
      | end
      | 
      | last = get_param(sys,'LastModifiedDate');
      | if isempty(last)
      |     last = datestr(now,'yyyy');
      | else
      |     last = last(end-3:end);
      | end
      | 
      | if strcmp(first,last)
      |     fprintf('%s -- Copyright %s Nexteer',NxtrConf,first)
      | else
      |     fprintf('%s -- %s%s- %s Nexteer',NxtrConf,char(169),first,last)
      | end
  RiseX : Outport
  RiseY : Outport  Port=2
  wires:
  PrevRiseX/1 -> RiseX/1
  PrevRiseY/1 -> RiseY/1

== system SF012A_HysCmp/HysCmp/HysCmpPer1/FilAndLimInp/CopyRight2 ==

== system SF012A_HysCmp/HysCmp/HysCmpPer1/FilAndLimInp/If Action Subsystem ==
  In1 : Inport
  In2 : Inport  Port=2
  Action Port : ActionPort  ActionType=then
  CopyRight2 : Subsystem  Description=|  mask(Copyright Information){none=on}
      | Copyright info block.                                               
      |                                                                     
      | Place copyright information at the top of every subsystem in design.
      mask prompts: none "No parameters"
      mask help: Place copyright information at the top of every subsystem in design.
      mask Display:
      | NxtrConf = 'Nexteer Confidential';
      | 
      | sys = bdroot; %handle for the current model ("system")
      | first = get_param(sys,'Created');
      | if(isempty(first))
      |     first = datestr(now,'yyyy');
      | else
      |     first = first(end-3:end);  %year is last four digits
      | end
      | 
      | last = get_param(sys,'LastModifiedDate');
      | if isempty(last)
      |     last = datestr(now,'yyyy');
      | else
      |     last = last(end-3:end);
      | end
      | 
      | if strcmp(first,last)
      |     fprintf('%s -- Copyright %s Nexteer',NxtrConf,first)
      | else
      |     fprintf('%s -- %s%s- %s Nexteer',NxtrConf,char(169),first,last)
      | end
  Out1 : Outport
  Out2 : Outport  Port=2
  wires:
  In1/1 -> Out1/1
  In2/1 -> Out2/1

== system SF012A_HysCmp/HysCmp/HysCmpPer1/FilAndLimInp/If Action Subsystem1 ==
  In1 : Inport
  In2 : Inport  Port=2
  Action Port : ActionPort  ActionType=else
  CopyRight2 : Subsystem  Description=|  mask(Copyright Information){none=on}
      | Copyright info block.                                               
      |                                                                     
      | Place copyright information at the top of every subsystem in design.
      mask prompts: none "No parameters"
      mask help: Place copyright information at the top of every subsystem in design.
      mask Display:
      | NxtrConf = 'Nexteer Confidential';
      | 
      | sys = bdroot; %handle for the current model ("system")
      | first = get_param(sys,'Created');
      | if(isempty(first))
      |     first = datestr(now,'yyyy');
      | else
      |     first = first(end-3:end);  %year is last four digits
      | end
      | 
      | last = get_param(sys,'LastModifiedDate');
      | if isempty(last)
      |     last = datestr(now,'yyyy');
      | else
      |     last = last(end-3:end);
      | end
      | 
      | if strcmp(first,last)
      |     fprintf('%s -- Copyright %s Nexteer',NxtrConf,first)
      | else
      |     fprintf('%s -- %s%s- %s Nexteer',NxtrConf,char(169),first,last)
      | end
  Out1 : Outport
  Out2 : Outport  Port=2
  wires:
  In1/1 -> Out1/1
  In2/1 -> Out2/1

== system SF012A_HysCmp/HysCmp/HysCmpPer1/FilHysCmpOutp/CopyRight2 ==

== system SF012A_HysCmp/HysCmp/HysCmpPer1/FilHysCmpOutp/HysCmp ==
  LpFilSts : Inport
  Action Port : ActionPort  ActionType=else
  Constant1 : Constant  Value=SysGlbPrmSysTqRat
  Constant2 : Constant  Value=HysCmpOutpLim
  CopyRight2 : Subsystem  Description=|  mask(Copyright Information){none=on}
      | Copyright info block.                                               
      |                                                                     
      | Place copyright information at the top of every subsystem in design.
      mask prompts: none "No parameters"
      mask help: Place copyright information at the top of every subsystem in design.
      mask Display:
      | NxtrConf = 'Nexteer Confidential';
      | 
      | sys = bdroot; %handle for the current model ("system")
      | first = get_param(sys,'Created');
      | if(isempty(first))
      |     first = datestr(now,'yyyy');
      | else
      |     first = first(end-3:end);  %year is last four digits
      | end
      | 
      | last = get_param(sys,'LastModifiedDate');
      | if isempty(last)
      |     last = datestr(now,'yyyy');
      | else
      |     last = last(end-3:end);
      | end
      | 
      | if strcmp(first,last)
      |     fprintf('%s -- Copyright %s Nexteer',NxtrConf,first)
      | else
      |     fprintf('%s -- %s%s- %s Nexteer',NxtrConf,char(169),first,last)
      | end
  FinalLim : NxtrLim/LimDyn_f32
  Product : Product  Inputs=*/  RndMeth=Zero
  Unary Minus2 : UnaryMinus
  Out : Outport
  wires:
  LpFilSts/1 -> FinalLim/1
  Unary Minus2/1 -> FinalLim/2
  Constant2/1 -> FinalLim/3, Unary Minus2/1
  FinalLim/1 -> Product/1
  Constant1/1 -> Product/2
  Product/1 -> Out/1

== system SF012A_HysCmp/HysCmp/HysCmpPer1/FilHysCmpOutp/Zero_Command ==
  Action Port : ActionPort  ActionType=then
  Constant1 : Constant  RequirementInfo={} %GIDa_058d0f85_193c_4c5a_9e4f_6786860596fd  Value=0  OutDataTypeStr=single
  CopyRight2 : Subsystem  Description=|  mask(Copyright Information){none=on}
      | Copyright info block.                                               
      |                                                                     
      | Place copyright information at the top of every subsystem in design.
      mask prompts: none "No parameters"
      mask help: Place copyright information at the top of every subsystem in design.
      mask Display:
      | NxtrConf = 'Nexteer Confidential';
      | 
      | sys = bdroot; %handle for the current model ("system")
      | first = get_param(sys,'Created');
      | if(isempty(first))
      |     first = datestr(now,'yyyy');
      | else
      |     first = first(end-3:end);  %year is last four digits
      | end
      | 
      | last = get_param(sys,'LastModifiedDate');
      | if isempty(last)
      |     last = datestr(now,'yyyy');
      | else
      |     last = last(end-3:end);
      | end
      | 
      | if strcmp(first,last)
      |     fprintf('%s -- Copyright %s Nexteer',NxtrConf,first)
      | else
      |     fprintf('%s -- %s%s- %s Nexteer',NxtrConf,char(169),first,last)
      | end
  Out : Outport
  wires:
  Constant1/1 -> Out/1

== system SF012A_HysCmp/HysCmp/HysCmpPer1/FltInj - Sim/CopyRight2 ==

== system SF012A_HysCmp/HysCmp/HysCmpPer1/CalcAvlCmp/CoulombFric/CopyRight2 ==

== system SF012A_HysCmp/HysCmp/HysCmpPer1/CalcRiseFac/LessCmp/CopyRight2 ==

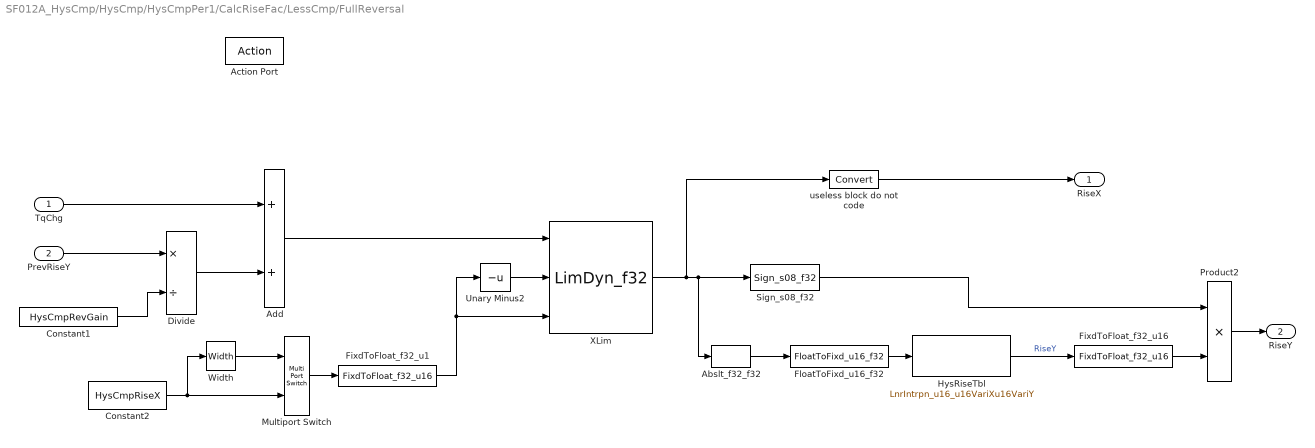
== system SF012A_HysCmp/HysCmp/HysCmpPer1/CalcRiseFac/LessCmp/FullReversal ==
  TqChg : Inport  RequirementInfo={'linktype_rmi_doors' '0000a52c (/E-STEER Core/SubSystem Specifications/Application Functions/SF012A Hysteresis Compensation)' '#SF012A_434' 'true' 'REQ:SF012A_434' '' } %GIDa_78511679_eeb3_40de_a8b0_557d994ee403
  PrevRiseY : Inport  RequirementInfo={'linktype_rmi_doors' '0000a52c (/E-STEER Core/SubSystem Specifications/Application Functions/SF012A Hysteresis Compensation)' '#SF012A_434' 'true' 'REQ:SF012A_434' '' } %GIDa_3d0132ad_cab3_4862_b472_f46cb3a6dc5f  Port=2
  Action Port : ActionPort  ActionType=else
  Abslt_f32_f32 : NxtrAbslt/Abslt_f32_f32  RequirementInfo={'linktype_rmi_doors' '0000a52c (/E-STEER Core/SubSystem Specifications/Application Functions/SF012A Hysteresis Compensation)' '#SF012A_436' 'true' 'REQ:SF012A_436' '' } %GIDa_2abae70f_df26_4108_b869_ffa99cf70fc6  SFunctionSpec=single y1 = Abslt_f32_f32(single u1)
      settings: AttributesFormatString=%<Name>
  Add : Sum  RequirementInfo={'linktype_rmi_doors' '0000a52c (/E-STEER Core/SubSystem Specifications/Application Functions/SF012A Hysteresis Compensation)' '#SF012A_434' 'true' 'REQ:SF012A_434' '' } %GIDa_51a01d6c_d6e7_4767_8f4c_e0c590b20aaa  RndMeth=Zero
  Constant1 : Constant  RequirementInfo={'linktype_rmi_doors' '0000a52c (/E-STEER Core/SubSystem Specifications/Application Functions/SF012A Hysteresis Compensation)' '#SF012A_434' 'true' 'REQ:SF012A_434' '' } %GIDa_82092ef1_6b01_4761_b7fb_dadcfa0a3c08  Value=HysCmpRevGain
  Constant2 : Constant  RequirementInfo={'linktype_rmi_doors' '0000a52c (/E-STEER Core/SubSystem Specifications/Application Functions/SF012A Hysteresis Compensation)' '#SF012A_435' 'true' 'REQ:SF012A_435' '' } %GIDa_3fd8485d_0e03_454a_a19b_46bc5cb93052  Value=HysCmpRiseX
  Divide : Product  RequirementInfo={'linktype_rmi_doors' '0000a52c (/E-STEER Core/SubSystem Specifications/Application Functions/SF012A Hysteresis Compensation)' '#SF012A_434' 'true' 'REQ:SF012A_434' '' } %GIDa_5f120b22_3b55_4951_a687_c3edf8196dfb  Inputs=*/  RndMeth=Zero
  FixdToFloat_f32_u1 : FixdToFloat/FixdToFloat_f32_u16  RequirementInfo={'linktype_rmi_doors' '0000a52c (/E-STEER Core/SubSystem Specifications/Application Functions/SF012A Hysteresis Compensation)' '#SF012A_435' 'true' 'REQ:SF012A_435' '' } %GIDa_fb32a101_9b4f_4d7d_9880_f7d8cb9bb6e3  Param1=14
  FixdToFloat_f32_u16 : FixdToFloat/FixdToFloat_f32_u16  RequirementInfo={'linktype_rmi_doors' '0000a52c (/E-STEER Core/SubSystem Specifications/Application Functions/SF012A Hysteresis Compensation)' '#SF012A_436' 'true' 'REQ:SF012A_436' '' } %GIDa_e9ff9a4f_f14b_40aa_9cc3_336a283a2f48  Param1=14
  FloatToFixd_u16_f32 : FloatToFixd/FloatToFixd_u16_f32  RequirementInfo={'linktype_rmi_doors' '0000a52c (/E-STEER Core/SubSystem Specifications/Application Functions/SF012A Hysteresis Compensation)' '#SF012A_436' 'true' 'REQ:SF012A_436' '' } %GIDa_5798adc7_cbae_4fe4_a219_6766996359af  Param1=14
  HysRiseTbl : LnrIntrpn/LnrIntrpn_u16_u16VariXu16VariY  RequirementInfo={'linktype_rmi_doors' '0000a52c (/E-STEER Core/SubSystem Specifications/Application Functions/SF012A Hysteresis Compensation)' '#SF012A_436' 'true' 'REQ:SF012A_436' '' } %GIDa_da3f9905_d23c_4be5_97a0_70a1107816c0  XTbl=HysCmpRiseX  YTbl=HysCmpRiseY
      settings: AttributesFormatString=Lnr ( u16VariX , u16VariY )
  Multiport Switch : MultiPortSwitch  RequirementInfo={'linktype_rmi_doors' '0000a52c (/E-STEER Core/SubSystem Specifications/Application Functions/SF012A Hysteresis Compensation)' '#SF012A_435' 'true' 'REQ:SF012A_435' '' } %GIDa_34b04f25_8256_46fe_8d1f_de8899ae5636  Inputs=1
  Product2 : Product  RequirementInfo={'linktype_rmi_doors' '0000a52c (/E-STEER Core/SubSystem Specifications/Application Functions/SF012A Hysteresis Compensation)' '#SF012A_436' 'true' 'REQ:SF012A_436' '' } %GIDa_049aeb9c_07d0_4acb_b762_5a9f45a80fb4  RndMeth=Zero
  Sign_s08_f32 : NxtrSign/Sign_s08_f32  RequirementInfo={'linktype_rmi_doors' '0000a52c (/E-STEER Core/SubSystem Specifications/Application Functions/SF012A Hysteresis Compensation)' '#SF012A_436' 'true' 'REQ:SF012A_436' '' } %GIDa_f6f70cd7_76a2_441a_9340_bc2899f3940a  SFunctionSpec=int8 y1 = Sign_s08_f32(single u1)
  Unary Minus2 : UnaryMinus  RequirementInfo={'linktype_rmi_doors' '0000a52c (/E-STEER Core/SubSystem Specifications/Application Functions/SF012A Hysteresis Compensation)' '#SF012A_435' 'true' 'REQ:SF012A_435' '' } %GIDa_c90906fd_46cf_4acb_9970_eb9ef222f842
  Width : Width  RequirementInfo={'linktype_rmi_doors' '0000a52c (/E-STEER Core/SubSystem Specifications/Application Functions/SF012A Hysteresis Compensation)' '#SF012A_435' 'true' 'REQ:SF012A_435' '' } %GIDa_b3f5525a_8b5e_41ee_bb01_7aff028a1c02  DataType=uint16
  XLim : NxtrLim/LimDyn_f32  RequirementInfo={'linktype_rmi_doors' '0000a52c (/E-STEER Core/SubSystem Specifications/Application Functions/SF012A Hysteresis Compensation)' '#SF012A_435' 'true' 'REQ:SF012A_435' '' } %GIDa_886358fd_52ae_49cf_8ae4_f398c961427d
  useless block do not code : DataTypeConversion
  RiseX : Outport
  RiseY : Outport  RequirementInfo={'linktype_rmi_doors' '0000a52c (/E-STEER Core/SubSystem Specifications/Application Functions/SF012A Hysteresis Compensation)' '#SF012A_436' 'true' 'REQ:SF012A_436' '' } %GIDa_b6f576a9_caa8_4012_b670_e6aa2d7b25f8  Port=2
  wires:
  Constant1/1 -> Divide/2
  PrevRiseY/1 -> Divide/1
  Divide/1 -> Add/2
  TqChg/1 -> Add/1
  Add/1 -> XLim/1
  FixdToFloat_f32_u1/1 -> XLim/3, Unary Minus2/1
  Unary Minus2/1 -> XLim/2
  XLim/1 -> Abslt_f32_f32/1, Sign_s08_f32/1, useless block do not code/1
  HysRiseTbl/1 -> FixdToFloat_f32_u16/1  "RiseY"
  Abslt_f32_f32/1 -> FloatToFixd_u16_f32/1
  Sign_s08_f32/1 -> Product2/1
  Product2/1 -> RiseY/1
  FixdToFloat_f32_u16/1 -> Product2/2
  FloatToFixd_u16_f32/1 -> HysRiseTbl/1
  Constant2/1 -> Multiport Switch/2, Width/1
  Width/1 -> Multiport Switch/1
  Multiport Switch/1 -> FixdToFloat_f32_u1/1
  useless block do not code/1 -> RiseX/1
